simulink model "model"  (R2021a)
settings: Solver=VariableStepAuto  StartTime=0.0  StopTime=100  RelTol=1e-3
undefined symbols (not defined in the file): DiscIntNeverNeededParam
libraries: simulink x12, fuzblock x6
settings Model: PacingRate=3  Creator=38095  LastModifiedBy=38095
settings SolverCC: ZeroCrossAlgorithm=Adaptive
settings DataIOCC: LimitDataPoints=on  SaveOutput=off  SaveTime=off
settings OptimizationCC: BlockReduction=off  BooleanDataType=off  LifeSpan=inf
settings DebuggingCC: SaveWithParameterizedLinksMsg=none  UnderspecifiedInitializationDetection=Classic  MergeDetectMultiDrivingBlocksExec=none  SignalResolutionControl=TryResolveAllWithWarning  IgnoredZcDiagnostic=none  AllowSymbolicDim=off  SFUnexpectedBacktrackingDiag=warning  SFNoUnconditionalDefaultTransitionDiag=warning  SFExecutionAtInitializationDiag=none  SFMachineParentedDataDiag=warning  UnderSpecifiedDimensionMsg=warning  ArithmeticOperatorsInVariantConditions=warning
settings HardwareCC: TargetUnknown=on
settings SFSimCC: SimUseLocalCustomCode=off  CustomCodeUndefinedFunction=UseInterfaceOnly
settings RTWCC: RTWUseLocalCustomCode=off
settings CodeAppCC: StateflowObjectComments=on
settings GRTTargetCC: TargetLangStandard=C89/C90 (ANSI)

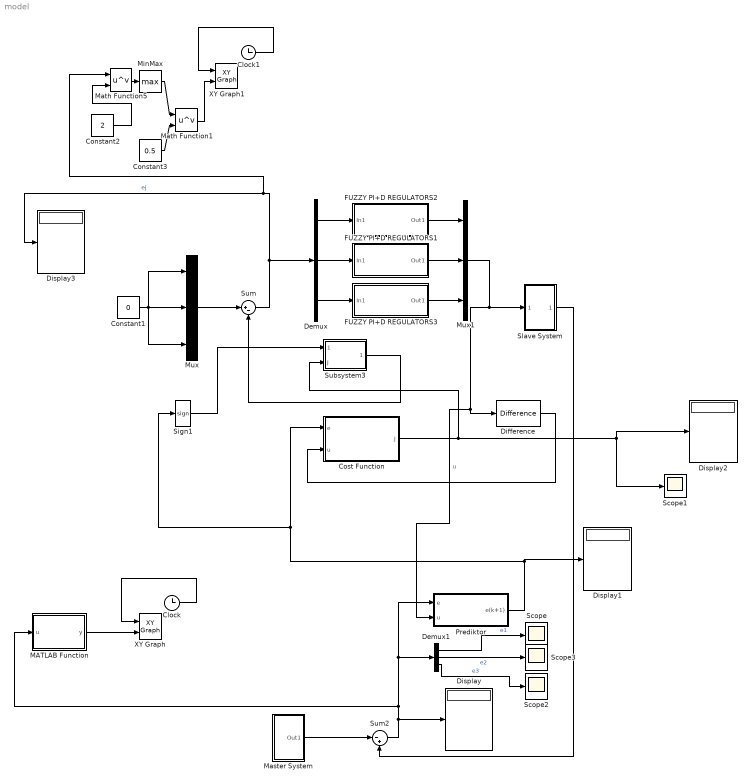
== system model ==
  Clock : Clock
  Clock1 : Clock
  Constant1 : Constant  Value=0
  Constant2 : Constant  Value=2
  Constant3 : Constant  Value=0.5
  Cost Function : Subsystem
  Demux : Demux  Outputs=3
  Demux1 : Demux  Outputs=3
  Difference : simulink/Discrete/Difference  ICPrevInput=0.0  OutMin=[]  OutMax=[]  OutDataType=fixdt(1, 16)  OutScaling=2^-10  DoSatur=off
  Display{,1..3} (4 alike) : Display
  FUZZY PI+D REGULATORS1 : Subsystem
  FUZZY PI+D REGULATORS2 : Subsystem
  FUZZY PI+D REGULATORS3 : Subsystem
  MATLAB Function : MATLAB Function  TreatAsAtomicUnit=on
  Master System : Subsystem
  Math Function1 : Math  Operator=pow  SaturateOnIntegerOverflow=on
  Math Function5 : Math  Operator=pow  SaturateOnIntegerOverflow=on
  MinMax : MinMax  Function=max
  Mux : Mux  Inputs=3
  Mux1 : Mux  Inputs=3
  Prediktor : Subsystem
  Scope{,1..3} (4 alike) : Scope
  Sign1 : Signum  ZeroCross=off
  Slave System : Subsystem
  Subsystem3 : Subsystem
  Sum : Sum  Inputs=|+-
  Sum2 : Sum  Inputs=|-+
  XY Graph : simulink/Sinks/XY Graph  xmin=0  xmax=100  ymin=0  ymax=100  st=-1
  XY Graph1 : simulink/Sinks/XY Graph  xmin=0  xmax=100  ymin=0  ymax=10000  st=-1
  wires:
  Master System/1(Out1) -> Sum2/1
  Slave System/1(Out3) -> Sum2/2
  Sum2/1 -> Demux1/1, Prediktor/1(e), MATLAB Function/1(u), Display/1
  Mux1/1 -> Slave System/1(In1), Prediktor/2(u), Difference/1  "u"
  Sign1/1 -> Subsystem3/1(Sign(e))
  Cost Function/1("J ") -> Subsystem3/2(J), Display2/1, Scope1/1
  Prediktor/1(e(k+1)) -> Sign1/1, Cost Function/1(e), Display1/1
  Mux/1 -> Sum/1
  Constant1/1 -> Mux/1, Mux/3, Mux/2
  Demux/1 -> FUZZY PI+D REGULATORS2/1(In1)
  Demux/2 -> FUZZY PI+D REGULATORS1/1(In1)
  Demux/3 -> FUZZY PI+D REGULATORS3/1(In1)
  FUZZY PI+D REGULATORS2/1(Out1) -> Mux1/1
  FUZZY PI+D REGULATORS1/1(Out1) -> Mux1/2
  FUZZY PI+D REGULATORS3/1(Out1) -> Mux1/3
  MATLAB Function/1(y) -> XY Graph/2
  Sum/1 -> Demux/1, Math Function5/1, Display3/1  "ej"
  Clock/1 -> XY Graph/1
  Clock1/1 -> XY Graph1/1
  Demux1/1 -> Scope/1  "e1"
  Demux1/2 -> Scope3/1  "e2"
  Demux1/3 -> Scope2/1  "e3"
  Math Function5/1 -> MinMax/1
  Constant2/1 -> Math Function5/2
  MinMax/1 -> Math Function1/1
  Constant3/1 -> Math Function1/2
  Math Function1/1 -> XY Graph1/2
  Difference/1 -> Cost Function/2(u)
  Subsystem3/1(Out1) -> Sum/2

== system model/Cost Function ==
  e : Inport
  u : Inport  Port=2
  Demux : Demux  Outputs=3
  Demux1 : Demux  Outputs=3
  Mux1 : Mux  Inputs=3
  Subsystem1 : Subsystem
  Subsystem2 : Subsystem
  Subsystem7 : Subsystem
  "J " : Outport
  wires:
  e/1 -> Demux/1
  u/1 -> Demux1/1
  Demux/1 -> Subsystem7/1(u)
  Demux1/1 -> Subsystem7/2(In2)
  Demux1/2 -> Subsystem1/2(In2)
  Demux1/3 -> Subsystem2/2(In2)
  Demux/3 -> Subsystem2/1(u)
  Subsystem7/1(Out1) -> Mux1/1
  Subsystem1/1(Out1) -> Mux1/2
  Subsystem2/1(Out1) -> Mux1/3
  Mux1/1 -> "J "/1
  Demux/2 -> Subsystem1/1(u)

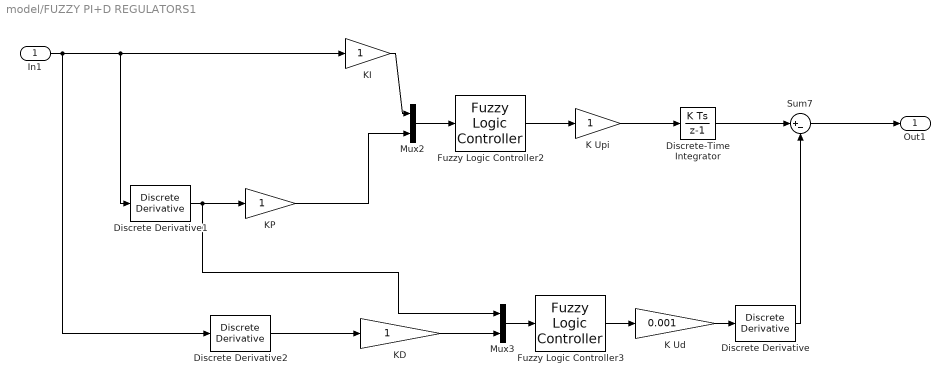
== system model/FUZZY PI+D REGULATORS1 ==
  In1 : Inport
  Discrete Derivative : simulink/Discrete/Discrete Derivative  gainval=1.0  ICPrevScaledInput=0.0  OutMin=[]  OutMax=[]  OutDataType=fixdt(1, 16)  OutScaling=2^-10  DoSatur=off
  Discrete Derivative1 : simulink/Discrete/Discrete Derivative  gainval=1.0  ICPrevScaledInput=0.0  OutMin=[]  OutMax=[]  OutDataType=fixdt(1, 16)  OutScaling=2^-10  DoSatur=off
  Discrete Derivative2 : simulink/Discrete/Discrete Derivative  gainval=1.0  ICPrevScaledInput=0.0  OutMin=[]  OutMax=[]  OutDataType=fixdt(1, 16)  OutScaling=2^-10  DoSatur=off
  Discrete-Time Integrator : DiscreteIntegrator  SampleTime=-1  ICPrevOutput=DiscIntNeverNeededParam  ICPrevScaledInput=DiscIntNeverNeededParam
  Fuzzy Logic Controller2 : fuzblock/Fuzzy Logic  Controller  FIS='FUZZY4.fis'  OutputSampleNumber=101  DataType=double  FuzzifiedInputs=off  RuleFiringStrengths=off  RuleOutputs=off  AggregatedOutputs=off  SimulateUsing=Interpreted execution  OutOfRangeInputValueMessage=warning  NoRuleFiredMessage=warning  EmptyOutputFuzzySetMessage=warning
  Fuzzy Logic Controller3 : fuzblock/Fuzzy Logic  Controller  FIS='FUZZY4.fis'  OutputSampleNumber=101  DataType=double  FuzzifiedInputs=off  RuleFiringStrengths=off  RuleOutputs=off  AggregatedOutputs=off  SimulateUsing=Interpreted execution  OutOfRangeInputValueMessage=warning  NoRuleFiredMessage=warning  EmptyOutputFuzzySetMessage=warning
  K Ud : Gain  Gain=0.001
  K Upi : Gain
  KD : Gain
  KI : Gain
  KP : Gain
  Mux2 : Mux  Inputs=2
  Mux3 : Mux  Inputs=2
  Sum7 : Sum  Inputs=|+-
  Out1 : Outport
  wires:
  KP/1 -> Mux2/2
  Mux2/1 -> Fuzzy Logic Controller2/1
  Fuzzy Logic Controller2/1 -> K Upi/1
  K Upi/1 -> Discrete-Time Integrator/1
  Discrete Derivative2/1 -> KD/1
  Mux3/1 -> Fuzzy Logic Controller3/1
  Fuzzy Logic Controller3/1 -> K Ud/1
  Sum7/1 -> Out1/1
  KD/1 -> Mux3/2
  KI/1 -> Mux2/1
  K Ud/1 -> Discrete Derivative/1
  Discrete Derivative1/1 -> Mux3/1, KP/1
  In1/1 -> Discrete Derivative2/1, Discrete Derivative1/1, KI/1
  Discrete-Time Integrator/1 -> Sum7/1
  Discrete Derivative/1 -> Sum7/2

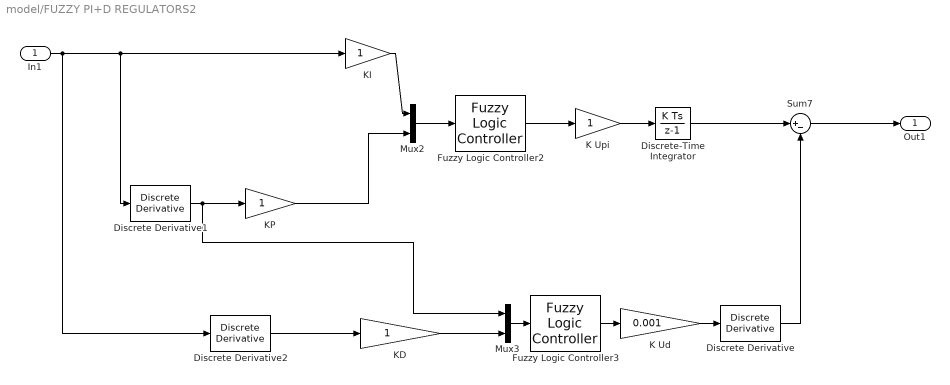
== system model/FUZZY PI+D REGULATORS2 ==
  In1 : Inport
  Discrete Derivative : simulink/Discrete/Discrete Derivative  gainval=1.0  ICPrevScaledInput=0.0  OutMin=[]  OutMax=[]  OutDataType=fixdt(1, 16)  OutScaling=2^-10  DoSatur=off
  Discrete Derivative1 : simulink/Discrete/Discrete Derivative  gainval=1.0  ICPrevScaledInput=0.0  OutMin=[]  OutMax=[]  OutDataType=fixdt(1, 16)  OutScaling=2^-10  DoSatur=off
  Discrete Derivative2 : simulink/Discrete/Discrete Derivative  gainval=1.0  ICPrevScaledInput=0.0  OutMin=[]  OutMax=[]  OutDataType=fixdt(1, 16)  OutScaling=2^-10  DoSatur=off
  Discrete-Time Integrator : DiscreteIntegrator  SampleTime=-1  ICPrevOutput=DiscIntNeverNeededParam  ICPrevScaledInput=DiscIntNeverNeededParam
  Fuzzy Logic Controller2 : fuzblock/Fuzzy Logic  Controller  FIS='FUZZY4.fis'  OutputSampleNumber=101  DataType=double  FuzzifiedInputs=off  RuleFiringStrengths=off  RuleOutputs=off  AggregatedOutputs=off  SimulateUsing=Interpreted execution  OutOfRangeInputValueMessage=warning  NoRuleFiredMessage=warning  EmptyOutputFuzzySetMessage=warning
  Fuzzy Logic Controller3 : fuzblock/Fuzzy Logic  Controller  FIS='FUZZY4.fis'  OutputSampleNumber=101  DataType=double  FuzzifiedInputs=off  RuleFiringStrengths=off  RuleOutputs=off  AggregatedOutputs=off  SimulateUsing=Interpreted execution  OutOfRangeInputValueMessage=warning  NoRuleFiredMessage=warning  EmptyOutputFuzzySetMessage=warning
  K Ud : Gain  Gain=0.001
  K Upi : Gain
  KD : Gain
  KI : Gain
  KP : Gain
  Mux2 : Mux  Inputs=2
  Mux3 : Mux  Inputs=2
  Sum7 : Sum  Inputs=|+-
  Out1 : Outport
  wires:
  KP/1 -> Mux2/2
  Mux2/1 -> Fuzzy Logic Controller2/1
  Fuzzy Logic Controller2/1 -> K Upi/1
  K Upi/1 -> Discrete-Time Integrator/1
  Discrete Derivative2/1 -> KD/1
  Mux3/1 -> Fuzzy Logic Controller3/1
  Fuzzy Logic Controller3/1 -> K Ud/1
  Sum7/1 -> Out1/1
  KD/1 -> Mux3/2
  KI/1 -> Mux2/1
  K Ud/1 -> Discrete Derivative/1
  Discrete Derivative1/1 -> Mux3/1, KP/1
  In1/1 -> Discrete Derivative2/1, Discrete Derivative1/1, KI/1
  Discrete-Time Integrator/1 -> Sum7/1
  Discrete Derivative/1 -> Sum7/2

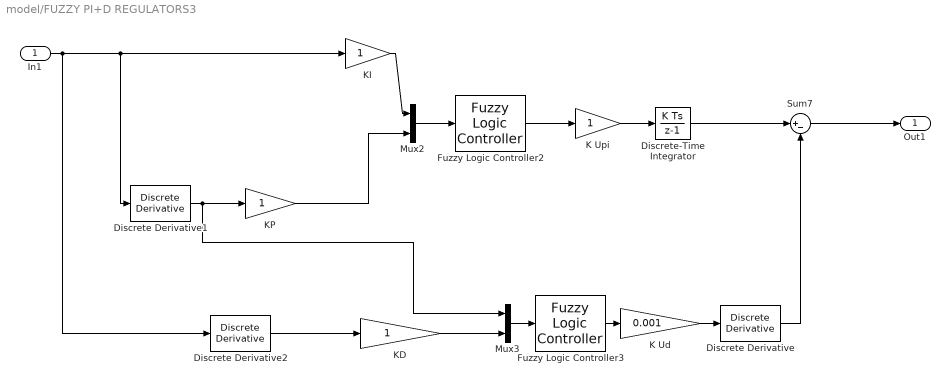
== system model/FUZZY PI+D REGULATORS3 ==
  In1 : Inport
  Discrete Derivative : simulink/Discrete/Discrete Derivative  gainval=1.0  ICPrevScaledInput=0.0  OutMin=[]  OutMax=[]  OutDataType=fixdt(1, 16)  OutScaling=2^-10  DoSatur=off
  Discrete Derivative1 : simulink/Discrete/Discrete Derivative  gainval=1.0  ICPrevScaledInput=0.0  OutMin=[]  OutMax=[]  OutDataType=fixdt(1, 16)  OutScaling=2^-10  DoSatur=off
  Discrete Derivative2 : simulink/Discrete/Discrete Derivative  gainval=1.0  ICPrevScaledInput=0.0  OutMin=[]  OutMax=[]  OutDataType=fixdt(1, 16)  OutScaling=2^-10  DoSatur=off
  Discrete-Time Integrator : DiscreteIntegrator  SampleTime=-1  ICPrevOutput=DiscIntNeverNeededParam  ICPrevScaledInput=DiscIntNeverNeededParam
  Fuzzy Logic Controller2 : fuzblock/Fuzzy Logic  Controller  FIS='FUZZY4.fis'  OutputSampleNumber=101  DataType=double  FuzzifiedInputs=off  RuleFiringStrengths=off  RuleOutputs=off  AggregatedOutputs=off  SimulateUsing=Interpreted execution  OutOfRangeInputValueMessage=warning  NoRuleFiredMessage=warning  EmptyOutputFuzzySetMessage=warning
  Fuzzy Logic Controller3 : fuzblock/Fuzzy Logic  Controller  FIS='FUZZY4.fis'  OutputSampleNumber=101  DataType=double  FuzzifiedInputs=off  RuleFiringStrengths=off  RuleOutputs=off  AggregatedOutputs=off  SimulateUsing=Interpreted execution  OutOfRangeInputValueMessage=warning  NoRuleFiredMessage=warning  EmptyOutputFuzzySetMessage=warning
  K Ud : Gain  Gain=0.001
  K Upi : Gain
  KD : Gain
  KI : Gain
  KP : Gain
  Mux2 : Mux  Inputs=2
  Mux3 : Mux  Inputs=2
  Sum7 : Sum  Inputs=|+-
  Out1 : Outport
  wires:
  KP/1 -> Mux2/2
  Mux2/1 -> Fuzzy Logic Controller2/1
  Fuzzy Logic Controller2/1 -> K Upi/1
  K Upi/1 -> Discrete-Time Integrator/1
  Discrete Derivative2/1 -> KD/1
  Mux3/1 -> Fuzzy Logic Controller3/1
  Fuzzy Logic Controller3/1 -> K Ud/1
  Sum7/1 -> Out1/1
  KD/1 -> Mux3/2
  KI/1 -> Mux2/1
  K Ud/1 -> Discrete Derivative/1
  Discrete Derivative1/1 -> Mux3/1, KP/1
  In1/1 -> Discrete Derivative2/1, Discrete Derivative1/1, KI/1
  Discrete-Time Integrator/1 -> Sum7/1
  Discrete Derivative/1 -> Sum7/2

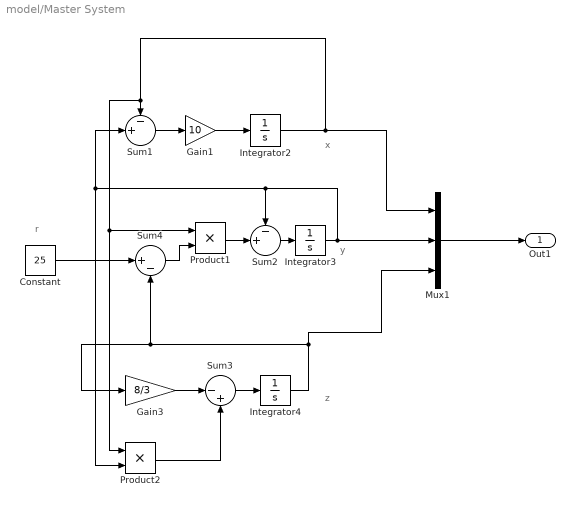
== system model/Master System ==
  note: x
  note: z
  note: y
  note: r
  Constant : Constant  Value=25
  Gain1 : Gain  Gain=10
  Gain3 : Gain  Gain=8/3
  Integrator2 : Integrator  InitialCondition=1  IgnoreLimit=on
  Integrator3 : Integrator  IgnoreLimit=on
  Integrator4 : Integrator  IgnoreLimit=on
  Mux1 : Mux  Inputs=3
  Product1 : Product
  Product2 : Product  InputSameDT=on
  Sum1 : Sum  Inputs=-+|
  Sum2 : Sum  Inputs=-+|
  Sum3 : Sum  Inputs=|-+
  Sum4 : Sum  Inputs=|+-
  Out1 : Outport
  wires:
  Gain3/1 -> Sum3/1
  Sum3/1 -> Integrator4/1
  Gain1/1 -> Integrator2/1
  Integrator3/1 -> Mux1/2, Sum1/2, Product2/2, Sum2/1
  Sum1/1 -> Gain1/1
  Integrator4/1 -> Mux1/3, Sum4/2, Gain3/1
  Product2/1 -> Sum3/2
  Sum4/1 -> Product1/2
  Product1/1 -> Sum2/2
  Integrator2/1 -> Mux1/1, Product2/1, Product1/1, Sum1/1
  Constant/1 -> Sum4/1
  Sum2/1 -> Integrator3/1
  Mux1/1 -> Out1/1

== system model/Prediktor ==
  e : Inport
  u : Inport  Port=2
  Demux : Demux  Outputs=3
  Demux1 : Demux  Outputs=3
  Mux1 : Mux  Inputs=3
  Subsystem1 : Subsystem
  Subsystem2 : Subsystem
  Subsystem6 : Subsystem
  e(k+1) : Outport
  wires:
  e/1 -> Demux/1
  u/1 -> Demux1/1
  Demux/1 -> Subsystem6/1(u)
  Demux1/1 -> Subsystem6/2(In2)
  Demux/2 -> Subsystem1/1(u)
  Demux1/2 -> Subsystem1/2(In2)
  Demux1/3 -> Subsystem2/2(In2)
  Demux/3 -> Subsystem2/1(u)
  Subsystem6/1(Out1) -> Mux1/1
  Subsystem1/1(Out1) -> Mux1/2
  Subsystem2/1(Out1) -> Mux1/3
  Mux1/1 -> e(k+1)/1

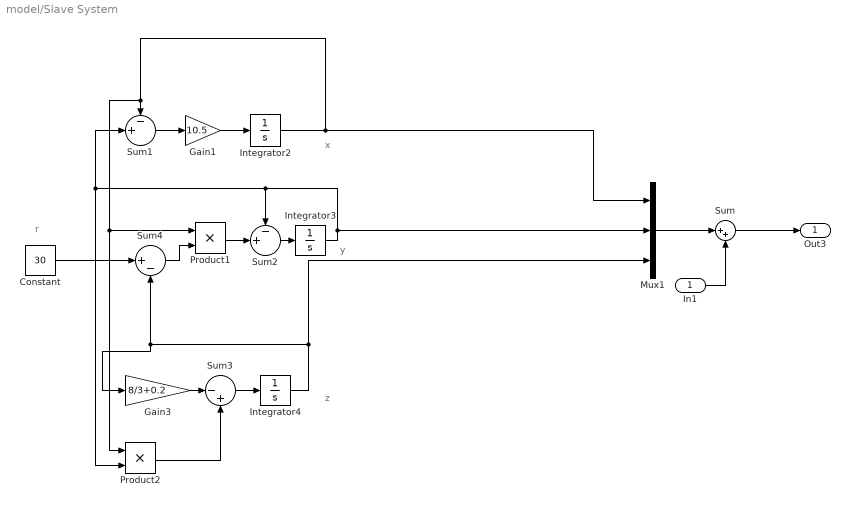
== system model/Slave System ==
  note: r
  note: y
  note: z
  note: x
  In1 : Inport
  Constant : Constant  Value=30
  Gain1 : Gain  Gain=10.5
  Gain3 : Gain  Gain=8/3+0.2
  Integrator2 : Integrator  InitialCondition=1  IgnoreLimit=on
  Integrator3 : Integrator  IgnoreLimit=on
  Integrator4 : Integrator  IgnoreLimit=on
  Mux1 : Mux  Inputs=3
  Product1 : Product
  Product2 : Product  InputSameDT=on
  Sum : Sum  Inputs=|++
  Sum1 : Sum  Inputs=-+|
  Sum2 : Sum  Inputs=-+|
  Sum3 : Sum  Inputs=|-+
  Sum4 : Sum  Inputs=|+-
  Out3 : Outport
  wires:
  Sum2/1 -> Integrator3/1
  Constant/1 -> Sum4/1
  Product1/1 -> Sum2/2
  Product2/1 -> Sum3/2
  Sum1/1 -> Gain1/1
  Sum4/1 -> Product1/2
  Sum3/1 -> Integrator4/1
  Gain1/1 -> Integrator2/1
  Gain3/1 -> Sum3/1
  Integrator4/1 -> Mux1/3, Sum4/2, Gain3/1
  Integrator3/1 -> Mux1/2, Sum1/2, Product2/2, Sum2/1
  Integrator2/1 -> Mux1/1, Product2/1, Product1/1, Sum1/1
  In1/1 -> Sum/2
  Mux1/1 -> Sum/1
  Sum/1 -> Out3/1

== system model/Subsystem3 ==
  Sign(e) : Inport
  J : Inport  Port=2
  Demux : Demux  Outputs=3
  Demux1 : Demux  Outputs=3
  Divide : Product  Inputs=**
  Divide1 : Product  Inputs=**
  Divide2 : Product  Inputs=**
  Mux : Mux  Inputs=3
  Out1 : Outport
  wires:
  Sign(e)/1 -> Demux/1
  J/1 -> Demux1/1
  Demux/1 -> Divide1/1
  Demux1/1 -> Divide1/2
  Demux/2 -> Divide/1
  Demux1/2 -> Divide/2
  Demux1/3 -> Divide2/2
  Demux/3 -> Divide2/1
  Mux/1 -> Out1/1
  Divide1/1 -> Mux/1
  Divide/1 -> Mux/2
  Divide2/1 -> Mux/3

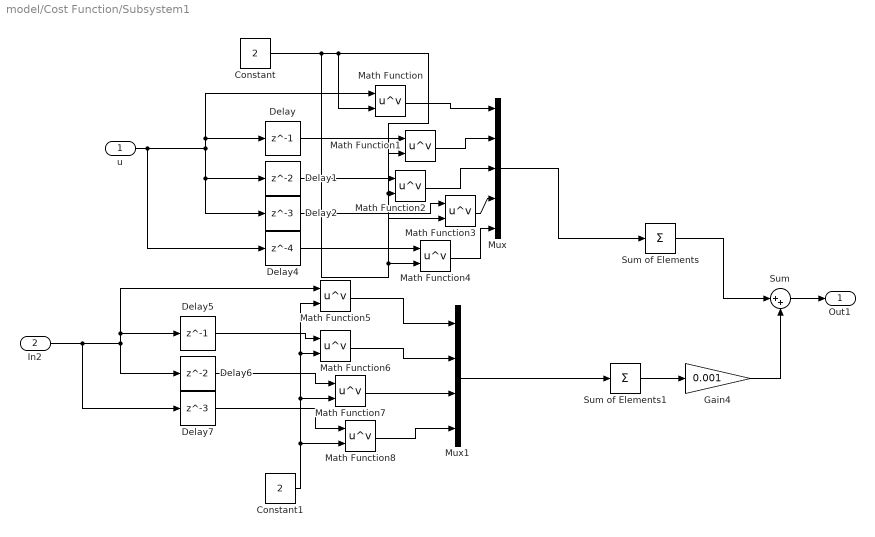
== system model/Cost Function/Subsystem1 ==
  u : Inport
  In2 : Inport  Port=2
  Constant : Constant  Value=2
  Constant1 : Constant  Value=2
  Delay : Delay  DelayLength=1
  Delay1 : Delay
  Delay2 : Delay  DelayLength=3
  Delay4 : Delay  DelayLength=4
  Delay5 : Delay  DelayLength=1
  Delay6 : Delay
  Delay7 : Delay  DelayLength=3
  Gain4 : Gain  Gain=0.001
  Math Function{,1..8} (9 alike) : Math  Operator=pow  SaturateOnIntegerOverflow=on
  Mux : Mux  Inputs=5
  Mux1 : Mux
  Sum : Sum  Inputs=|++
  Sum of Elements : Sum  Inputs=+
  Sum of Elements1 : Sum  Inputs=+
  Out1 : Outport
  wires:
  Mux/1 -> Sum of Elements/1
  Constant/1 -> Math Function3/2, Math Function/2, Math Function4/2, Math Function2/2, Math Function1/2
  u/1 -> Delay4/1, Math Function/1, Delay/1, Delay2/1, Delay1/1
  Math Function/1 -> Mux/1
  Delay/1 -> Math Function1/1
  Math Function1/1 -> Mux/2
  Delay1/1 -> Math Function2/1
  Math Function2/1 -> Mux/3
  Delay2/1 -> Math Function3/1
  Math Function3/1 -> Mux/4
  Delay4/1 -> Math Function4/1
  In2/1 -> Delay7/1, Math Function5/1, Delay5/1, Delay6/1
  Math Function5/1 -> Mux1/1
  Delay5/1 -> Math Function6/1
  Math Function6/1 -> Mux1/2
  Delay6/1 -> Math Function7/1
  Math Function7/1 -> Mux1/3
  Delay7/1 -> Math Function8/1
  Constant1/1 -> Math Function7/2, Math Function6/2, Math Function5/2, Math Function8/2
  Mux1/1 -> Sum of Elements1/1
  Sum of Elements1/1 -> Gain4/1
  Gain4/1 -> Sum/2
  Sum of Elements/1 -> Sum/1
  Sum/1 -> Out1/1
  Math Function8/1 -> Mux1/4
  Math Function4/1 -> Mux/5

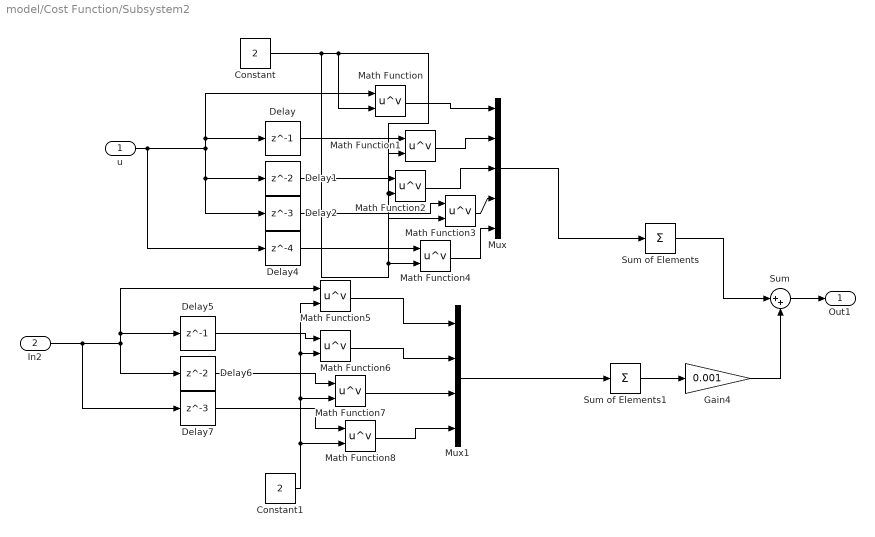
== system model/Cost Function/Subsystem2 ==
  u : Inport
  In2 : Inport  Port=2
  Constant : Constant  Value=2
  Constant1 : Constant  Value=2
  Delay : Delay  DelayLength=1
  Delay1 : Delay
  Delay2 : Delay  DelayLength=3
  Delay4 : Delay  DelayLength=4
  Delay5 : Delay  DelayLength=1
  Delay6 : Delay
  Delay7 : Delay  DelayLength=3
  Gain4 : Gain  Gain=0.001
  Math Function{,1..8} (9 alike) : Math  Operator=pow  SaturateOnIntegerOverflow=on
  Mux : Mux  Inputs=5
  Mux1 : Mux
  Sum : Sum  Inputs=|++
  Sum of Elements : Sum  Inputs=+
  Sum of Elements1 : Sum  Inputs=+
  Out1 : Outport
  wires:
  Mux/1 -> Sum of Elements/1
  Constant/1 -> Math Function3/2, Math Function/2, Math Function4/2, Math Function2/2, Math Function1/2
  u/1 -> Delay4/1, Math Function/1, Delay/1, Delay2/1, Delay1/1
  Math Function/1 -> Mux/1
  Delay/1 -> Math Function1/1
  Math Function1/1 -> Mux/2
  Delay1/1 -> Math Function2/1
  Math Function2/1 -> Mux/3
  Delay2/1 -> Math Function3/1
  Math Function3/1 -> Mux/4
  Delay4/1 -> Math Function4/1
  In2/1 -> Delay7/1, Math Function5/1, Delay5/1, Delay6/1
  Math Function5/1 -> Mux1/1
  Delay5/1 -> Math Function6/1
  Math Function6/1 -> Mux1/2
  Delay6/1 -> Math Function7/1
  Math Function7/1 -> Mux1/3
  Delay7/1 -> Math Function8/1
  Constant1/1 -> Math Function7/2, Math Function6/2, Math Function5/2, Math Function8/2
  Mux1/1 -> Sum of Elements1/1
  Sum of Elements1/1 -> Gain4/1
  Gain4/1 -> Sum/2
  Sum of Elements/1 -> Sum/1
  Sum/1 -> Out1/1
  Math Function8/1 -> Mux1/4
  Math Function4/1 -> Mux/5

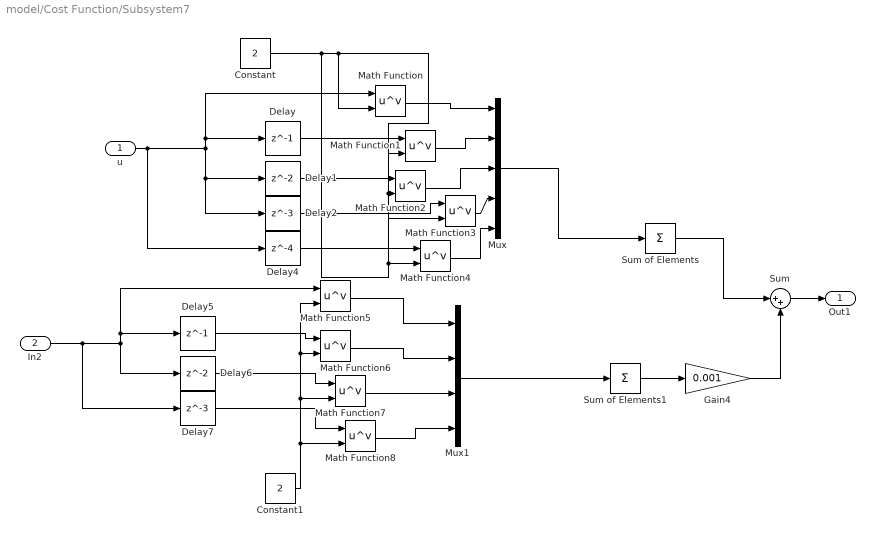
== system model/Cost Function/Subsystem7 ==
  u : Inport
  In2 : Inport  Port=2
  Constant : Constant  Value=2
  Constant1 : Constant  Value=2
  Delay : Delay  DelayLength=1
  Delay1 : Delay
  Delay2 : Delay  DelayLength=3
  Delay4 : Delay  DelayLength=4
  Delay5 : Delay  DelayLength=1
  Delay6 : Delay
  Delay7 : Delay  DelayLength=3
  Gain4 : Gain  Gain=0.001
  Math Function{,1..8} (9 alike) : Math  Operator=pow  SaturateOnIntegerOverflow=on
  Mux : Mux  Inputs=5
  Mux1 : Mux
  Sum : Sum  Inputs=|++
  Sum of Elements : Sum  Inputs=+
  Sum of Elements1 : Sum  Inputs=+
  Out1 : Outport
  wires:
  Mux/1 -> Sum of Elements/1
  Constant/1 -> Math Function3/2, Math Function/2, Math Function4/2, Math Function2/2, Math Function1/2
  u/1 -> Delay4/1, Math Function/1, Delay/1, Delay2/1, Delay1/1
  Math Function/1 -> Mux/1
  Delay/1 -> Math Function1/1
  Math Function1/1 -> Mux/2
  Delay1/1 -> Math Function2/1
  Math Function2/1 -> Mux/3
  Delay2/1 -> Math Function3/1
  Math Function3/1 -> Mux/4
  Delay4/1 -> Math Function4/1
  In2/1 -> Delay7/1, Math Function5/1, Delay5/1, Delay6/1
  Math Function5/1 -> Mux1/1
  Delay5/1 -> Math Function6/1
  Math Function6/1 -> Mux1/2
  Delay6/1 -> Math Function7/1
  Math Function7/1 -> Mux1/3
  Delay7/1 -> Math Function8/1
  Constant1/1 -> Math Function7/2, Math Function6/2, Math Function5/2, Math Function8/2
  Mux1/1 -> Sum of Elements1/1
  Sum of Elements1/1 -> Gain4/1
  Gain4/1 -> Sum/2
  Sum of Elements/1 -> Sum/1
  Sum/1 -> Out1/1
  Math Function8/1 -> Mux1/4
  Math Function4/1 -> Mux/5

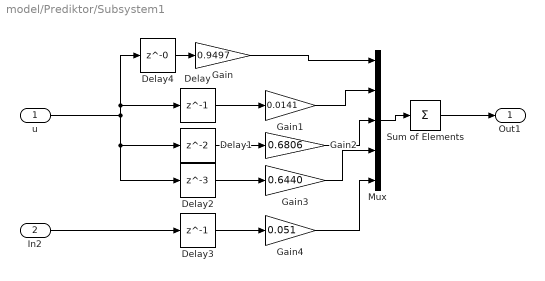
== system model/Prediktor/Subsystem1 ==
  u : Inport
  In2 : Inport  Port=2
  Delay : Delay  DelayLength=1
  Delay1 : Delay
  Delay2 : Delay  DelayLength=3
  Delay3 : Delay  DelayLength=1
  Delay4 : Delay  DelayLength=0  InitialCondition=5
  Gain : Gain  Gain=0.9497
  Gain1 : Gain  Gain=0.0141
  Gain2 : Gain  Gain=0.6806
  Gain3 : Gain  Gain=0.6440
  Gain4 : Gain  Gain=0.051
  Mux : Mux  Inputs=5
  Sum of Elements : Sum  Inputs=+
  Out1 : Outport
  wires:
  Gain/1 -> Mux/1
  Mux/1 -> Sum of Elements/1
  Delay/1 -> Gain1/1
  Gain1/1 -> Mux/2
  Delay1/1 -> Gain2/1
  Gain2/1 -> Mux/3
  u/1 -> Delay/1, Delay4/1, Delay2/1, Delay1/1
  Delay2/1 -> Gain3/1
  Gain3/1 -> Mux/4
  In2/1 -> Delay3/1
  Gain4/1 -> Mux/5
  Delay3/1 -> Gain4/1
  Sum of Elements/1 -> Out1/1
  Delay4/1 -> Gain/1

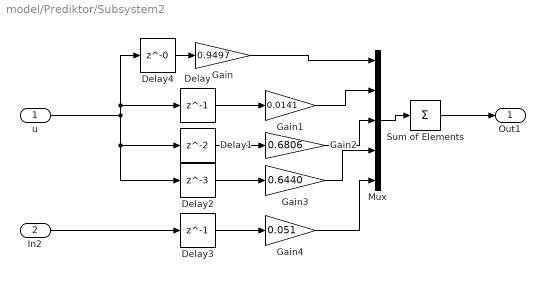
== system model/Prediktor/Subsystem2 ==
  u : Inport
  In2 : Inport  Port=2
  Delay : Delay  DelayLength=1
  Delay1 : Delay
  Delay2 : Delay  DelayLength=3
  Delay3 : Delay  DelayLength=1
  Delay4 : Delay  DelayLength=0  InitialCondition=-7
  Gain : Gain  Gain=0.9497
  Gain1 : Gain  Gain=0.0141
  Gain2 : Gain  Gain=0.6806
  Gain3 : Gain  Gain=0.6440
  Gain4 : Gain  Gain=0.051
  Mux : Mux  Inputs=5
  Sum of Elements : Sum  Inputs=+
  Out1 : Outport
  wires:
  Gain/1 -> Mux/1
  Mux/1 -> Sum of Elements/1
  Delay/1 -> Gain1/1
  Gain1/1 -> Mux/2
  Delay1/1 -> Gain2/1
  Gain2/1 -> Mux/3
  u/1 -> Delay/1, Delay4/1, Delay2/1, Delay1/1
  Delay2/1 -> Gain3/1
  Gain3/1 -> Mux/4
  In2/1 -> Delay3/1
  Gain4/1 -> Mux/5
  Delay3/1 -> Gain4/1
  Sum of Elements/1 -> Out1/1
  Delay4/1 -> Gain/1

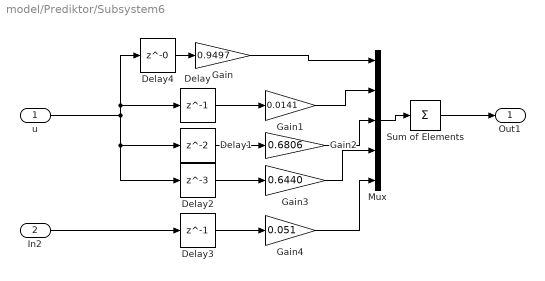
== system model/Prediktor/Subsystem6 ==
  u : Inport
  In2 : Inport  Port=2
  Delay : Delay  DelayLength=1
  Delay1 : Delay
  Delay2 : Delay  DelayLength=3
  Delay3 : Delay  DelayLength=1
  Delay4 : Delay  DelayLength=0
  Gain : Gain  Gain=0.9497
  Gain1 : Gain  Gain=0.0141
  Gain2 : Gain  Gain=0.6806
  Gain3 : Gain  Gain=0.6440
  Gain4 : Gain  Gain=0.051
  Mux : Mux  Inputs=5
  Sum of Elements : Sum  Inputs=+
  Out1 : Outport
  wires:
  Gain/1 -> Mux/1
  Mux/1 -> Sum of Elements/1
  Delay/1 -> Gain1/1
  Gain1/1 -> Mux/2
  Delay1/1 -> Gain2/1
  Gain2/1 -> Mux/3
  u/1 -> Delay/1, Delay4/1, Delay2/1, Delay1/1
  Delay2/1 -> Gain3/1
  Gain3/1 -> Mux/4
  In2/1 -> Delay3/1
  Gain4/1 -> Mux/5
  Delay3/1 -> Gain4/1
  Sum of Elements/1 -> Out1/1
  Delay4/1 -> Gain/1

== matlab function model/MATLAB Function ==
  data: u input; y output
function y = fcn(u)
x=0;
for i=1:length(u)
    x=x+u(i).^2;
end
y = x.^(1/2);
